simulink model "FirstOrderSystem"  (R2023b)
settings: Solver=VariableStepAuto  StartTime=0.0  StopTime=20  RelTol=1e-3
values from neighbouring files (symbols this model uses):
  G4_den = [a b]    [FirstOrderSystem_PlantWithTimeDelay.m]
  G4_num = A    (= 1)    [FirstOrderSystem_PlantWithTimeDelay.m]
settings Model: Creator=Zolo  LastModifiedBy=Zolo

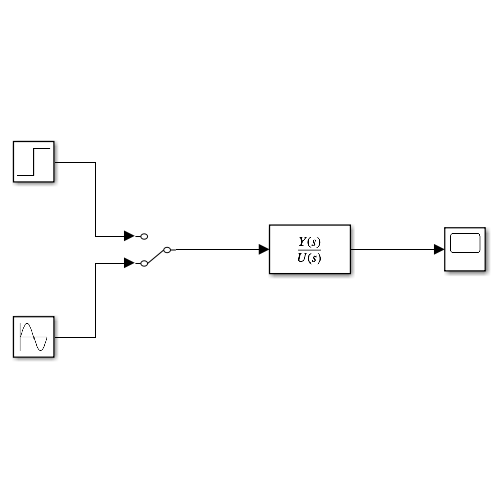
[thumbnail: Simulink's stored preview of the top-level diagram]
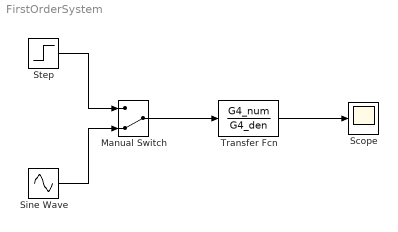
== system FirstOrderSystem ==
  Manual Switch : ManualSwitch  CurrentSetting=0
  Scope : Scope
  Sine Wave : Sin  SampleTime=0
  Step : Step  SampleTime=0
  Transfer Fcn : TransferFcn  Numerator=G4_num  Denominator=G4_den
  wires:
  Step/1 -> Manual Switch/1
  Sine Wave/1 -> Manual Switch/2
  Manual Switch/1 -> Transfer Fcn/1
  Transfer Fcn/1 -> Scope/1
